simulink model "DFT_Stream_Ex1"  (R2023a)
settings: Solver=VariableStepAuto  StartTime=0.0  StopTime=1  RelTol=1e-3
undefined symbols (not defined in the file): None, S, vsva2197, xcvc1902
libraries: aieUtilities x2, dspsrcs4 x1, aieDSP x1, vmcUtilities x1
settings Model: Creator=sdegala  LastModifiedBy=robg
settings ModelReferenceCC: EnableRefExpFcnMdlSchedulingChecks=on

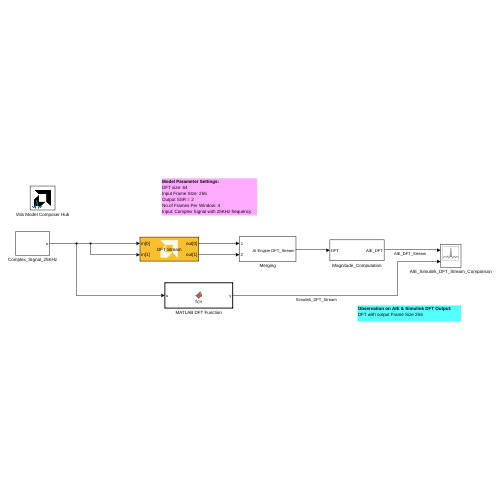
[thumbnail: Simulink's stored preview of the top-level diagram]
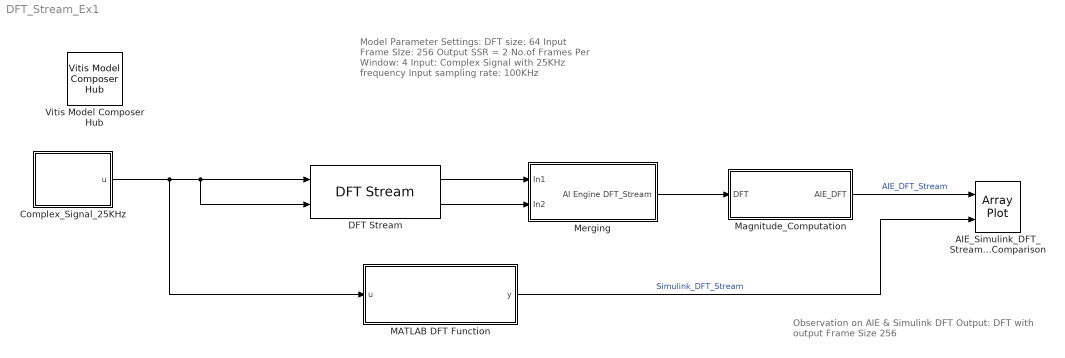
== system DFT_Stream_Ex1 ==
  note: Model Parameter Settings:
      | DFT size: 64
      | Input Frame SIze: 256
      | Output SSR = 2
      | No.of Frames Per Window: 4
      | Input: Complex Signal with 25KHz frequency
      | Input sampling rate: 100KHz
  note: Observation on AIE & Simulink DFT Output:
      | DFT with output Frame Size 256
  AIE_Simulink_DFT_Stream_Comparison : ArrayPlot  NumInputPorts=2  WindowPosition=[215.000000,122.000000,845.000000,423.000000,]  Visible=on  ScopeFrameLocation=window  YLimits=[-80,720]  ShowLegend=on
  Complex_Signal_25KHz : Subsystem
  DFT Stream : aieDSP/DFT Stream  data_type=cfloat  twiddle_type=cfloat  point_size=64  num_frames=4  shift_val=0  rnd_mode=Round symmetrical to infinity  ssr=2  sat_mode=0-None  casc_length=1  AIE_VARIANT=1  blockJsonConstraints=[]  blockJsonConstraintsInternal=[]  spec=vmc_stream_dft.json  SerializedMaskParamNames=[]  SerializedMaskParamValues=[]  SerializedMaskParamVisibilities=[]  block_type=DFT Stream  SerializedMaskParamDataypes=typename|typename|uint|uint|uint|uint|uint|uint|uint|uint  SerializedMaskParamEnumStrArr=0|0|0|0|0|Floor,Ceiling,Round to positive infinity,Round to negative infinity,Round symmetrical to infinity,Round symmetrical to zero,Round convergent to even,Round convergent to odd|0|0-None,1-Asymmetric,3-Symmetric|0|0  SerializedMaskParamEnumValArr=0|0|0|0|0|0,1,2,3,4,5,6,7|0|0,1,3|0|0  SerializedMaskParamVectorArr=0|0|0|0|0|0|0|0|0|0
  MATLAB DFT Function : MATLAB Function  TreatAsAtomicUnit=on
  Magnitude_Computation : Subsystem
  Merging : Subsystem
  Vitis Model Composer Hub : vmcUtilities/Vitis Model Composer Hub  Tag=genX  CodeGeneration=off  StartColumn=1  NumberOfColumns=1  TargetDirectory=./code  exportDesign=off  analyzeDesign=off  validateDesignOnHw=off  ExportType=AI Engines  IpVendor=xilinx.com  IpLibrary=hls  IpVersion=1.0  IpHWLanguage=Verilog  AieCompilerOptions={}  AieSimulatorOptions={}  CreateTestbench=off  TestbenchStackSize=10  RunRtlSim=off  RunCSim=off  RunAieSim=off  AieSimTimeout=50000  RunAieSimProfiling=off  LaunchVitisAnalyzer=off  PlotOutput=off  RunX86Sim=off  X86SimTimeout=10  GenHwImage=off  GenLibadfXo=off  GenHwValidationCode=off  PlatformType=Not Specified  HwSystemType=Baremetal  HwValidationTarget=hw  ProjDevice=xcvc1902-vsva2197-1LP-e-S  ProjDevicePart=xcvc1902-vsva2197-1LP-e-S  AIEType=AIE  SamplePeriod=-1  ClockFrequency=200  DataPathParallelism=1  xilinxfamily=versalaicore  part=xcvc1902  speed=-1LP-e-S  package=vsva2197  directory=./code  testbench=off  incr_netlist=off  synthesis_tool=Vivado  clock_wrapper=Clock Enables  dbl_ovrd=According to Block Masks  dcm_input_clock_period=10  sysclk_period=10  simulink_period=1  eval_field=0  LogFileName=''  NThreads=4
  wires:
  Merging/1(AI Engine DFT_Stream) -> Magnitude_Computation/1(DFT)
  MATLAB DFT Function/1(y) -> AIE_Simulink_DFT_Stream_Comparison/2  "Simulink_DFT_Stream"
  Complex_Signal_25KHz/1(u) -> DFT Stream/2, DFT Stream/1, MATLAB DFT Function/1(u)
  DFT Stream/1 -> Merging/1(In1)
  DFT Stream/2 -> Merging/2(In2)
  Magnitude_Computation/1(AIE_DFT) -> AIE_Simulink_DFT_Stream_Comparison/1  "AIE_DFT_Stream"

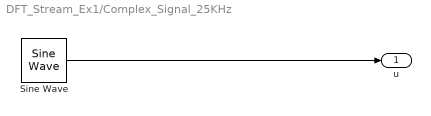
== system DFT_Stream_Ex1/Complex_Signal_25KHz ==
  Sine Wave : dspsrcs4/Sine Wave  Amplitude=10  Frequency=25e3  Phase=0  SampleMode=Discrete  OutComplex=Complex  CompMethod=Table lookup  TableSize=Speed  SampleTime=1/100e3  SamplesPerFrame=256  ResetState=Restart at time zero  OutputFrames=off  dataType=single  wordLen=16  udDataType=sfix(16)  fracBitsMode=User-defined  numFracBits=10  OutDataTypeStr=single  LastOutDataTypeStr=single
  u : Outport
  wires:
  Sine Wave/1 -> u/1

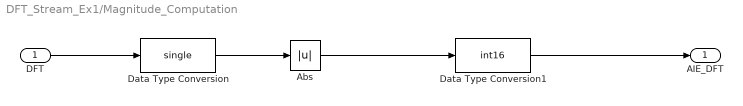
== system DFT_Stream_Ex1/Magnitude_Computation ==
  DFT : Inport
  Abs : Abs  SaturateOnIntegerOverflow=off
  Data Type Conversion : DataTypeConversion  OutDataTypeStr=single  SaturateOnIntegerOverflow=off  RndMeth=Floor
  Data Type Conversion1 : DataTypeConversion  OutDataTypeStr=int16  SaturateOnIntegerOverflow=off  RndMeth=Floor
  AIE_DFT : Outport
  wires:
  Data Type Conversion/1 -> Abs/1
  DFT/1 -> Data Type Conversion/1
  Abs/1 -> Data Type Conversion1/1
  Data Type Conversion1/1 -> AIE_DFT/1

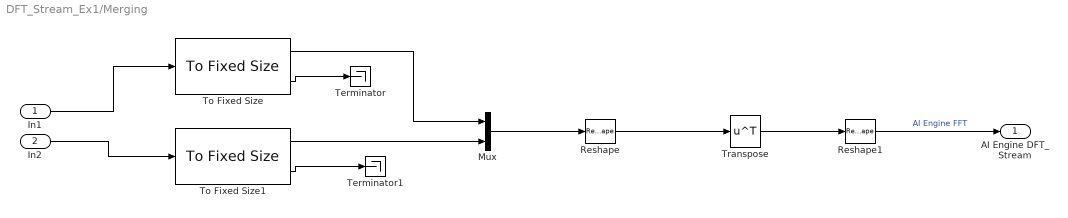
== system DFT_Stream_Ex1/Merging ==
  In1 : Inport
  In2 : Inport  Port=2
  Mux : Mux  Inputs=2
  Reshape : Reshape  OutputDimensionality=Customize  OutputDimensions=[128, 2]
  Reshape1 : Reshape  OutputDimensions=[1, 10]
  Terminator : Terminator
  Terminator1 : Terminator
  To Fixed Size : aieUtilities/To Fixed Size  Mode=Produce a valid output signal  OutputSize=Inherit: Same as input  CopyMethod=Buffer samples to form output  HasStatusOutput=on
  To Fixed Size1 : aieUtilities/To Fixed Size  Mode=Produce a valid output signal  OutputSize=Inherit: Same as input  CopyMethod=Buffer samples to form output  HasStatusOutput=on
  Transpose : Math  Operator=transpose
  AI Engine DFT_Stream : Outport
  wires:
  Reshape/1 -> Transpose/1
  To Fixed Size1/2 -> Terminator1/1
  To Fixed Size1/1 -> Mux/2
  In2/1 -> To Fixed Size1/1
  To Fixed Size/2 -> Terminator/1
  Transpose/1 -> Reshape1/1
  To Fixed Size/1 -> Mux/1
  Mux/1 -> Reshape/1
  Reshape1/1 -> AI Engine DFT_Stream/1  "AI Engine FFT"
  In1/1 -> To Fixed Size/1

== matlab function DFT_Stream_Ex1/MATLAB DFT Function ==
  data: u input; y output

function y = fcn(u)

DFT_Size = 64; % DFT Size
FramesPerWindow = 4; %No.of Frames Per Window


X = single(complex(zeros(DFT_Size,FramesPerWindow)));

for m = 1:1:FramesPerWindow
for k = 0:DFT_Size-1
    for n = 0:DFT_Size-1
        X(k+1,m) = X(k+1,m) + u(n+1)*exp(-1i*2*pi*n*k/DFT_Size);
    end
end
end

y = abs(reshape(X,DFT_Size*FramesPerWindow,1));
